simulink model "gm_commrshdl"  (R2023b)
settings: Solver=FixedStepDiscrete  StartTime=0.0  StopTime=21000  RelTol=1e-3
libraries: hdlsllib x2, whdlutilities x2, simulink x1, simulink_extras x1, whdledac x1
settings Model: ModifiedByFormat=The MathWorks Inc.  Creator=The MathWorks, Inc.  LastModifiedBy=The MathWorks Inc.
settings SolverCC: AlgebraicLoopSolver=TrustRegion
settings DataIOCC: LimitDataPoints=on  SaveFormat=Array  SaveOutput=off  SaveTime=off  ReturnWorkspaceOutputs=off  SignalLoggingName=RS_HDL_logsout
settings OptimizationCC: BlockReduction=off  ConditionallyExecuteInputs=off  DefaultParameterBehavior=Inlined  InheritOutputTypeSmallerThanSingle=on  ExpressionDepthLimit=2147483647  LifeSpan=inf
settings DebuggingCC: AlgebraicLoopMsg=error  UnderspecifiedInitializationDetection=Classic  MergeDetectMultiDrivingBlocksExec=none  SolverPrmCheckMsg=warning  InheritedTsInSrcMsg=none  MultiTaskDSMMsg=warning  MultiTaskCondExecSysMsg=none  SingleTaskRateTransMsg=error  UnconnectedInputMsg=warning  UnconnectedOutputMsg=warning  UnconnectedLineMsg=warning  AllowSymbolicDim=off  StateNameClashWarn=warning  SymbolicDimsDataTypeCodeGenerationDiagnostic=none  SFUnexpectedBacktrackingDiag=warning  SFNoUnconditionalDefaultTransitionDiag=warning  SFExecutionAtInitializationDiag=none  ArithmeticOperatorsInVariantConditions=warning
settings HardwareCC: ProdBitPerPointer=32  ProdBitPerSizeT=32  ProdBitPerPtrDiffT=32  ProdLargestAtomicFloat=None  ProdIntDivRoundTo=Undefined  ProdEndianess=Unspecified  ProdWordSize=32  ProdHWDeviceType=ASIC/FPGA->ASIC/FPGA  ProdEqTarget=off
settings ModelReferenceCC: EnableRefExpFcnMdlSchedulingChecks=on  PropagateSignalLabelsOutOfModel=off
settings SFSimCC: SimUseLocalCustomCode=off  CustomCodeUndefinedFunction=UseInterfaceOnly
settings RTWCC: RTWUseLocalCustomCode=off
settings CodeAppCC: StateflowObjectComments=on
settings GRTTargetCC: TargetLangStandard=C89/C90 (ANSI)
settings ConfigComp: CovMetricSettings=dw  CovSaveCumulativeToWorkspaceVar=on  CovSaveSingleToWorkspaceVar=on  CovExternalEMLEnable=off  CovSFcnEnable=off

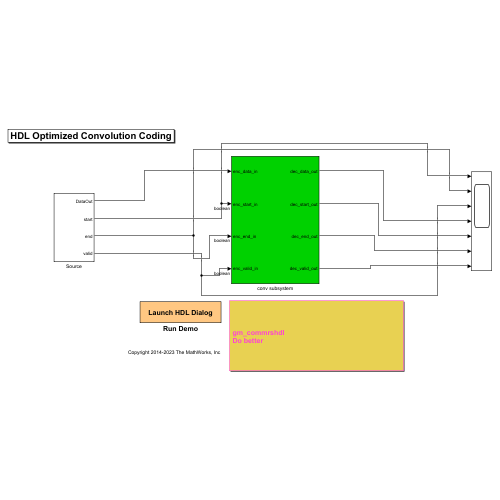
[thumbnail: Simulink's stored preview of the top-level diagram]
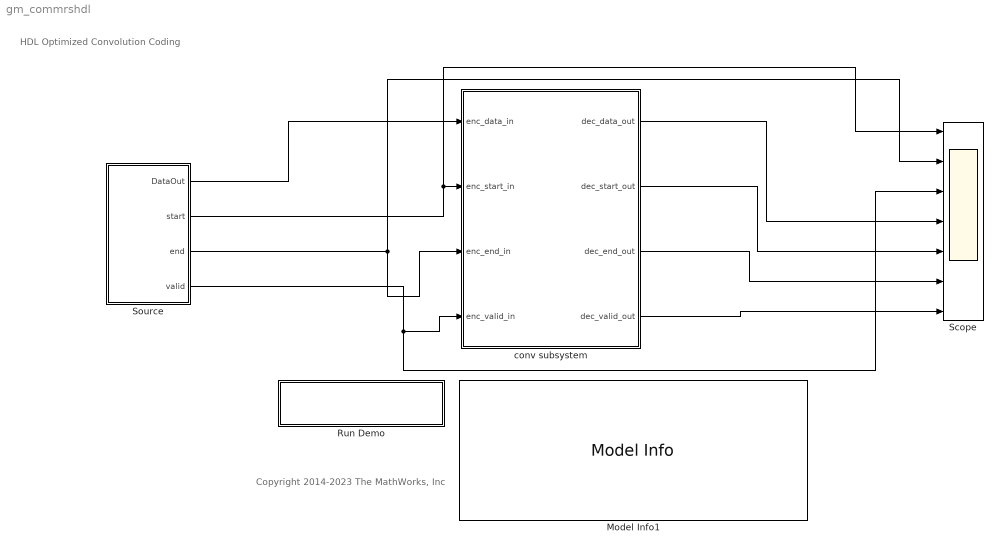
== system gm_commrshdl ==
  note: Copyright 2014-2023 The MathWorks, Inc
  note: HDL Optimized Convolution Coding
  Model Info1 : simulink/Model-Wide Utilities/Model Info  Frame=on  DisplayStringWithTags=|  HorizontalTextAlignment=Left  LeftAlignmentValue=0.02
      | %<ModelName>
      | Do better
  Run Demo : Subsystem
      settings: OpenFcn=hdldialog(bdroot)
      mask Display: disp('Launch HDL Dialog')
  Scope : Scope  NumInputPorts=7
  Source : Subsystem
  conv subsystem : Subsystem
  wires:
  Source/2(start) -> conv subsystem/2(enc_start_in), Scope/1
  Source/3(end) -> conv subsystem/3(enc_end_in), Scope/2
  Source/4(valid) -> conv subsystem/4(enc_valid_in), Scope/3
  conv subsystem/1(dec_data_out) -> Scope/4
  conv subsystem/4(dec_valid_out) -> Scope/7
  conv subsystem/3(dec_end_out) -> Scope/6
  conv subsystem/2(dec_start_out) -> Scope/5
  Source/1(DataOut) -> conv subsystem/1(enc_data_in)

== system gm_commrshdl/Run Demo ==

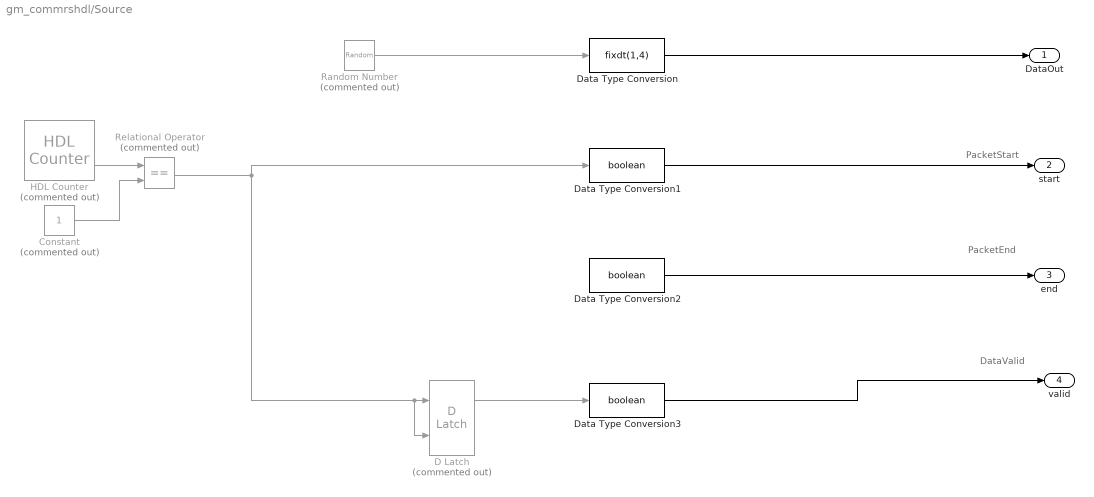
== system gm_commrshdl/Source ==
  note: PacketStart
  note: PacketEnd
  note: DataValid
  Constant : Constant  Commented=on
  D Latch : simulink_extras/Flip Flops/D Latch  Commented=on
  Data Type Conversion : DataTypeConversion  OutMin=[0]  OutMax=[65335]  OutDataTypeStr=fixdt(1,4)  SaturateOnIntegerOverflow=off  RndMeth=Floor  LockScale=on
  Data Type Conversion1 : DataTypeConversion  OutDataTypeStr=boolean  SaturateOnIntegerOverflow=off  RndMeth=Floor
  Data Type Conversion2 : DataTypeConversion  OutDataTypeStr=boolean  SaturateOnIntegerOverflow=off  RndMeth=Floor
  Data Type Conversion3 : DataTypeConversion  OutDataTypeStr=boolean  SaturateOnIntegerOverflow=off  RndMeth=Floor
  HDL Counter : hdlsllib/Sources/HDL Counter  Commented=on  CountType=Count limited  CountInit=0  CountStep=1  CountMax=3  CountFromType=Initial value  CountFrom=0  CountResetPort=off  CountLoadPort=off  CountEnbPort=off  CountDirPort=off  CountHitOutputPort=on  CountDataType=Unsigned  CountWordLen=8  CountFracLen=0  CountSampTime=1
  Random Number : RandomNumber  Commented=on  SampleTime=0.1
  Relational Operator : RelationalOperator  Commented=on  Operator===  OutDataTypeStr=boolean  InputSameDT=off
  DataOut : Outport  VectorParamsAs1DForOutWhenUnconnected=off
  start : Outport  Port=2  VectorParamsAs1DForOutWhenUnconnected=off
  end : Outport  Port=3  VectorParamsAs1DForOutWhenUnconnected=off
  valid : Outport  Port=4  VectorParamsAs1DForOutWhenUnconnected=off
  wires:
  Data Type Conversion1/1 -> start/1
  Data Type Conversion2/1 -> end/1
  Data Type Conversion/1 -> DataOut/1
  Data Type Conversion3/1 -> valid/1
  D Latch/1 -> Data Type Conversion3/1
  Random Number/1 -> Data Type Conversion/1
  Relational Operator/1 -> D Latch/2, D Latch/1, Data Type Conversion1/1
  ? -> Data Type Conversion2/1
  HDL Counter/2 -> Relational Operator/1
  Constant/1 -> Relational Operator/2

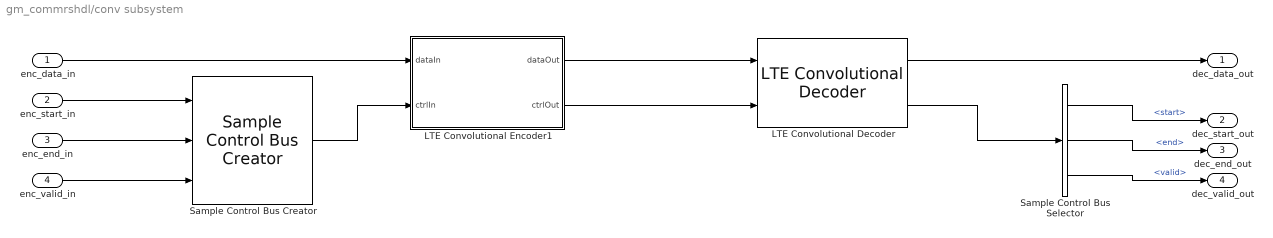
== system gm_commrshdl/conv subsystem ==
  enc_data_in : Inport
  enc_start_in : Inport  Port=2  OutDataTypeStr=boolean
  enc_end_in : Inport  Port=3  OutDataTypeStr=boolean
  enc_valid_in : Inport  Port=4  OutDataTypeStr=boolean
  LTE Convolutional Decoder : whdledac/LTE Convolutional Decoder  MaximumMessageLength=1024  SimulateUsing=Code generation
  LTE Convolutional Encoder1 : Subsystem  AncestorBlock=whdledac/LTE Convolutional Encoder  mask(LTE Convolutional Encoder){BuffSize=1024}
      mask prompts: BuffSize "Maximum message length"
      mask help:
      | Implements a tailbiting convolutional encoder with the following parameters:
      | Rate 1/3
      | Constraint length 7
      | Octal code generator [133, 171, 165]
      mask init:
      | ltehdl.internal.ConvEncoderInit(gcb);
      mask DialogControl DescGroupVar Prompt: LTE Convolutional Encoder
      mask DialogControl DescTextVar Prompt: Implements a tailbiting convolutional encoder with the following parameters:
      mask DialogControl DescTextVar_copy Prompt: Rate 1/3
      mask DialogControl DescTextVar_copy_copy Prompt: Constraint length 7
      mask DialogControl DescTextVar_copy_copy_copy Prompt: Octal code generator [133, 171, 165]
      mask Display:
      | disp('LTE Convolutional\nEncoder');
      | port_label('input',1,'data');
      | port_label('input',2,'ctrl');
      | port_label('output',1,'data');
      | port_label('output',2,'ctrl');
  Sample Control Bus Creator : whdlutilities/Sample Control Bus Creator
  Sample Control Bus Selector : whdlutilities/Sample Control Bus Selector  OutputSignals=start,end,valid
  dec_data_out : Outport  VectorParamsAs1DForOutWhenUnconnected=off
  dec_start_out : Outport  Port=2  VectorParamsAs1DForOutWhenUnconnected=off
  dec_end_out : Outport  Port=3  VectorParamsAs1DForOutWhenUnconnected=off
  dec_valid_out : Outport  Port=4  VectorParamsAs1DForOutWhenUnconnected=off
  wires:
  LTE Convolutional Encoder1/2(ctrlOut) -> LTE Convolutional Decoder/2
  LTE Convolutional Encoder1/1(dataOut) -> LTE Convolutional Decoder/1
  Sample Control Bus Selector/3 -> dec_valid_out/1  "<valid>"
  Sample Control Bus Selector/2 -> dec_end_out/1  "<end>"
  Sample Control Bus Selector/1 -> dec_start_out/1  "<start>"
  LTE Convolutional Decoder/1 -> dec_data_out/1
  LTE Convolutional Decoder/2 -> Sample Control Bus Selector/1
  Sample Control Bus Creator/1 -> LTE Convolutional Encoder1/2(ctrlIn)
  enc_data_in/1 -> LTE Convolutional Encoder1/1(dataIn)
  enc_valid_in/1 -> Sample Control Bus Creator/3
  enc_end_in/1 -> Sample Control Bus Creator/2
  enc_start_in/1 -> Sample Control Bus Creator/1

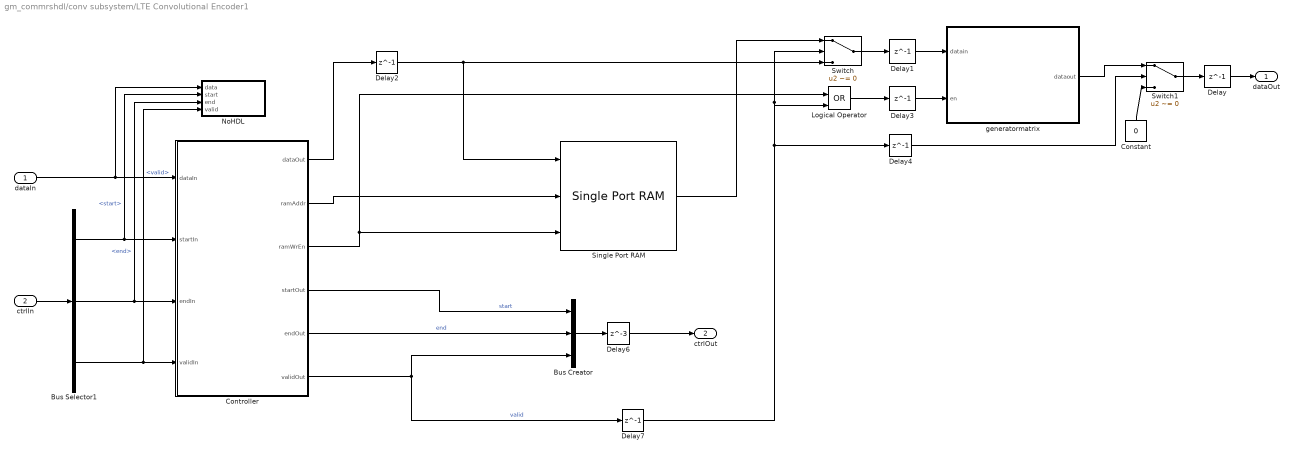
== system gm_commrshdl/conv subsystem/LTE Convolutional Encoder1 ==
  dataIn : Inport
  ctrlIn : Inport  Port=2
  Bus Creator : BusCreator  Inputs=3  OutDataTypeStr=Bus: samplecontrol  NonVirtualBus=on
      mask init:
      | registersamplecontrolbus;
      settings: InheritFromInputs=off
  Bus Selector1 : BusSelector  OutputSignals=start,end,valid
  Constant : Constant  Value=0  OutDataTypeStr=boolean  SampleTime=-1
  Controller : MATLAB Function  TreatAsAtomicUnit=on
  Delay : Delay  DelayLength=1
  Delay1 : Delay  DelayLength=1
  Delay2 : Delay  DelayLength=1  InitialCondition=0  UseCircularBuffer=on
  Delay3 : Delay  DelayLength=1
  Delay4 : Delay  DelayLength=1  InitialCondition=0  UseCircularBuffer=on
  Delay6 : Delay  DelayLength=3  InitialCondition=0  UseCircularBuffer=on
  Delay7 : Delay  DelayLength=1  InitialCondition=0  UseCircularBuffer=on
  Logical Operator : Logic  Operator=OR  IconShape=distinctive  AllPortsSameDT=off  OutDataTypeStr=boolean
  NoHDL : Subsystem
  Single Port RAM : hdlsllib/HDL RAMs/Single Port RAM  ram_size=nextpow2(BuffSize)  dout_type=Old data
  Switch : Switch  Criteria=u2 ~= 0  SaturateOnIntegerOverflow=off  InputSameDT=off
  Switch1 : Switch  Criteria=u2 ~= 0  SaturateOnIntegerOverflow=off  InputSameDT=off
  generatormatrix : MATLAB Function  TreatAsAtomicUnit=on
  dataOut : Outport  VectorParamsAs1DForOutWhenUnconnected=off
  ctrlOut : Outport  Port=2  VectorParamsAs1DForOutWhenUnconnected=off
  wires:
  Switch1/1 -> Delay/1
  dataIn/1 -> Controller/1(dataIn), NoHDL/1(data)
  Bus Creator/1 -> Delay6/1
  Controller/2(ramAddr) -> Single Port RAM/2
  Bus Selector1/2 -> Controller/3(endIn), NoHDL/3(end)  "<end>"
  Delay/1 -> dataOut/1
  Controller/4(startOut) -> Bus Creator/1  "start"
  Controller/5(endOut) -> Bus Creator/2  "end"
  Bus Selector1/3 -> Controller/4(validIn), NoHDL/4(valid)  "<valid>"
  Delay2/1 -> Single Port RAM/1, Switch/3
  ctrlIn/1 -> Bus Selector1/1
  Controller/3(ramWrEn) -> Single Port RAM/3, Logical Operator/1
  Logical Operator/1 -> Delay3/1
  Bus Selector1/1 -> Controller/2(startIn), NoHDL/2(start)  "<start>"
  Delay1/1 -> generatormatrix/1(datain)
  Delay4/1 -> Switch1/2
  generatormatrix/1(dataout) -> Switch1/1
  Controller/1(dataOut) -> Delay2/1
  Constant/1 -> Switch1/3
  Delay3/1 -> generatormatrix/2(en)
  Controller/6(validOut) -> Delay7/1, Bus Creator/3  "valid"
  Switch/1 -> Delay1/1
  Delay6/1 -> ctrlOut/1
  Delay7/1 -> Delay4/1, Switch/2, Logical Operator/2
  Single Port RAM/1 -> Switch/1

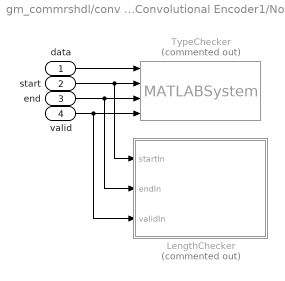
== system gm_commrshdl/conv subsystem/LTE Convolutional Encoder1/NoHDL ==
  data : Inport
  start : Inport  Port=2
  end : Inport  Port=3
  valid : Inport  Port=4
  LengthChecker : MATLAB Function  Commented=on  TreatAsAtomicUnit=on
  TypeChecker : MATLABSystem  Commented=on  System=ltehdl.internal.ConvEncCheckType  SimulateUsing=Code generation
      mask Type: ltehdl.internal.ConvEncCheckType
      mask Display: disp('ConvEncCheckType');
  wires:
  valid/1 -> TypeChecker/4, LengthChecker/3(validIn)
  start/1 -> TypeChecker/2, LengthChecker/1(startIn)
  data/1 -> TypeChecker/1
  end/1 -> TypeChecker/3, LengthChecker/2(endIn)

== matlab function gm_commrshdl/conv subsystem/LTE Convolutional Encoder1/Controller ==
  settings: fimath=fimath('RoundingMethod', 'Floor','OverflowAction', 'Wrap','ProductMode', 'FullPrecision', 'SumMode', 'FullPrecision')
  data: dataIn input; dataOut output; startIn input; ramAddr output; endIn input; validIn input; ramWrEn output; startOut output; endOut output; validOut output; BuffSize parameter double
function [dataOut, ramAddr, ramWrEn, startOut, endOut, validOut] = Controller(dataIn,startIn,endIn,validIn, BuffSize)
    %#codegen
    
    % states
    ENC_IDLE          = 0;        % waiting for start
    ENC_STREAM_IN     = 1;        % streaming input and writing into RAM
    ENC_STREAM_IN_END = 2;        % last input bit
    ENC_STREAM_OUT    = 3;        % stream data out of RAM through encoder
    
    persistent encoderStateReg;   % current state of decoder
    persistent ramAddrReg;        % buffer write address
    persistent ramAddrEndReg;     % value at which rd_addr counter should stop counting
    persistent ramWrEnReg;        % buffer write enable
    persistent dataReg;
    
    if isempty(ramWrEnReg)
        encoderStateReg = fi(ENC_IDLE,0,2,0);
        ramAddrReg      = fi(0,0,nextpow2(BuffSize),0,'OverflowAction','Wrap');
        ramAddrEndReg   = fi(0,0,nextpow2(BuffSize),0,'OverflowAction','Wrap');
        ramWrEnReg      = false;
        if isa(dataIn,'embedded.fi')
            dataReg = fi(false(length(dataIn),1),dataIn.numerictype); %ufi(0,1,0);
        else
            dataReg = cast(zeros(length(dataIn),1),class(dataIn));
        end
    end
    
    % assign outputs
    if nextpow2(BuffSize) == 8
        ramAddr       = uint8(ramAddrReg);
    elseif nextpow2(BuffSize) == 16
        ramAddr       = uint16(ramAddrReg);
    else
        ramAddr       = ramAddrReg;
    end
    ramWrEn       = ramWrEnReg;
    startOut      = (encoderStateReg == ENC_STREAM_OUT) && (ramAddrReg == 0);
    endOut        = (encoderStateReg == ENC_STREAM_OUT) && (ramAddrReg == ramAddrEndReg);
    validOut      = (encoderStateReg == ENC_STREAM_OUT);
    %     ready         = (encoderStateReg == ENC_IDLE);
    
    %----------------------------------------------------------------------------------------------
    % synchronous logic
    %----------------------------------------------------------------------------------------------
    
    ramWrEnReg(:) = validIn && (startIn || (encoderStateReg == ENC_STREAM_IN));
    
    if (encoderStateReg == ENC_STREAM_IN_END)
        ramAddrEndReg(:) = ramAddrReg;
    end
    
    switch encoderStateReg
        case ENC_IDLE
            
            if validIn && startIn
                encoderStateReg(:) = ENC_STREAM_IN;
                ramAddrReg(:)      = 0;
            end
            
        case ENC_STREAM_IN
            
            if validIn
                if endIn
                    encoderStateReg(:) = ENC_STREAM_IN_END;
                    ramAddrReg(:)      = ramAddrReg + 1;
                elseif startIn
                    encoderStateReg(:) = ENC_STREAM_IN;
                    ramAddrReg(:) = 0;
                else
                    encoderStateReg(:) = ENC_STREAM_IN;
                    ramAddrReg(:)      = ramAddrReg + 1;
                end
            end
            
        case ENC_STREAM_IN_END
            
            %             encoderStateReg(:) = ENC_STREAM_OUT;
            ramAddrReg(:)      = 0;
            if validIn && startIn
                encoderStateReg(:) = ENC_STREAM_IN;
            else
                encoderStateReg(:) = ENC_STREAM_OUT;
            end
            
        case ENC_STREAM_OUT
            
            if validIn && startIn
                ramAddrReg(:) = 0;
                encoderStateReg(:) = ENC_STREAM_IN;
            else
                if (ramAddrReg == ramAddrEndReg)
                    encoderStateReg(:) = ENC_IDLE;
                    ramAddrReg(:)      = 0;
                else
                    encoderStateReg(:) = ENC_STREAM_OUT;
                    ramAddrReg(:)      = ramAddrReg + 1;
                end
            end
    end
    
    dataReg(:) = dataIn;
    dataOut = dataIn(1);
    
end

== matlab function gm_commrshdl/conv subsystem/LTE Convolutional Encoder1/generatormatrix ==
  settings: fimath=fimath('RoundingMethod', 'Floor','OverflowAction', 'Wrap','ProductMode', 'FullPrecision', 'SumMode', 'FullPrecision')
  data: dataIn input; dataOut output; en input
function dataOut  = FunctionGenerator(dataIn,en)
    %#codegen
    
    G_value = [...
        1 0 1 1 0 1 1;
        1 1 1 1 0 0 1;
        1 1 1 0 1 0 1];
    
    localFimath = fimath(...
        'OverflowAction', 'Wrap', ...
        'ProductMode', 'SpecifyPrecision', ...
        'ProductWordLength', 1, ...
        'ProductFractionLength', 0, ...
        'SumMode', 'SpecifyPrecision', ...
        'SumWordLength', 1, ...
        'SumFractionLength', 0);
    
    G = fi(G_value, 0, 1, 0, localFimath);
    
    % current state of decoder
    persistent shiftReg;
    
    if isempty(shiftReg)
        shiftReg = fi(zeros(7,1), 0, 1, 0, localFimath);
    end
    
    % shift register
    shiftRegNext = shiftReg;
    if en
        shiftRegNext = [cast(dataIn,'like',shiftReg); shiftReg(1:6)];
    end
    
    % compute function output
    dataOut = G * shiftRegNext;
    
    shiftReg = shiftRegNext;
    
end

== matlab function gm_commrshdl/conv subsystem/LTE Convolutional Encoder1/NoHDL/LengthChecker ==
  settings: fimath=fimath('RoundingMethod', 'Floor','OverflowAction', 'Wrap','ProductMode', 'FullPrecision', 'SumMode', 'FullPrecision')
  data: startIn input; endIn input; validIn input; BuffSize parameter
function checkMsgLength(startIn,endIn,validIn, BuffSize)
    % Check the length of frame if matches the LTE standard.
    
    WAIT_S = ufi(0,2,0);
    COUNT_S = ufi(1,2,0);
    RST_S = ufi(2,2,0);
    
    persistent lenState;
    persistent lenCounter;
    
    if isempty(lenState)
        lenState= WAIT_S;
        lenCounter = ufi(0,17,0);
    end
    
    nextLenState   = lenState;
    nextLenCounter = lenCounter;
    
    switch(lenState)
        case WAIT_S
            nextLenCounter(:) = 0;
            if startIn && validIn
                nextLenState = COUNT_S;
            else
                nextLenState = WAIT_S;
            end
            
        case COUNT_S
            if validIn
                if endIn
                    nextLenCounter(:) = lenCounter + 1;
                    nextLenState = RST_S;
                elseif startIn
                    nextLenCounter(:) = 0;
                else
                    nextLenCounter(:) = lenCounter + 1;
                end
            end
        otherwise
            if validIn && startIn
                nextLenState = COUNT_S;
                nextLenCounter(:) = 0;
            else
                nextLenState = WAIT_S;
            end
    end
    
    if (nextLenCounter <5 || nextLenCounter > BuffSize-1) && (endIn == true) && nextLenState == RST_S
        coder.internal.warning('whdl:ConvolutionalCode:InvalidDataLength',int2str(double(nextLenCounter+1)));
    end
    
    lenState   = nextLenState;
    lenCounter = nextLenCounter;
    
end
